simulink model "fixed_point_pi_local_q"  (R2023b)
settings: Solver=FixedStepDiscrete  StartTime=0.0  StopTime=0.02  FixedStep=5.0000000000000002e-05  RelTol=1e-3
values from neighbouring files (symbols this model uses):
  Ki_dt_local = Ki_local * Ts    (= 0.005)    [build_fixed_point_pi_local_q_model.m]
  Kp_local = 10    [build_fixed_point_pi_local_q_model.m]
  Ts = 0.00005    (= 5e-05)    [build_fixed_point_pi_local_q_model.m]    (also in build_fixed_point_pi_q14_model.m)
  Umax_local = 1.8    [build_fixed_point_pi_local_q_model.m]
  Umin_local = -1.8    [build_fixed_point_pi_local_q_model.m]
settings Model: Creator=user  LastModifiedBy=user
settings OptimizationCC: DefaultParameterBehavior=Inlined  EnhancedBackFolding=on  PassReuseOutputArgsAs=Individual arguments  ZeroExternalMemoryAtStartup=off  ZeroInternalMemoryAtStartup=off  OptimizeBlockOrder=speed  DifferentSizesBufferReuse=on  OptimizationCustomize=off  EfficientTunableParamExpr=on
settings DebuggingCC: ParameterTunabilityLossMsg=error
settings HardwareCC: ProdBitPerPointer=32  ProdBitPerSizeT=32  ProdBitPerPtrDiffT=32  ProdLargestAtomicInteger=Long  ProdLargestAtomicFloat=Double  ProdWordSize=32  ProdHWDeviceType=ARM Compatible->ARM Cortex  TargetLargestAtomicInteger=Long  TargetLargestAtomicFloat=Double  TargetIntDivRoundTo=Zero  TargetEndianess=LittleEndian  TargetHWDeviceType=ARM Compatible->ARM Cortex  ProdEqTarget=off
settings SFSimCC: MATLABDynamicMemAlloc=off
settings RTWCC: Description=Embedded Coder  SystemTargetFile=ert.tlc  GenCodeOnly=on  TemplateMakefile=ert_default_tmf  GenerateReport=on
settings CodeAppCC: ForceParamTrailComments=on  IgnoreCustomStorageClasses=off  OperatorAnnotations=on  SimulinkDataObjDesc=on  SFDataObjDesc=on  InsertBlockDesc=on
settings ERTTargetCC: TargetLangStandard=C99 (ISO)  GenerateSampleERTMain=on  InlinedParameterPlacement=NonHierarchical  ERTCustomFileTemplate=example_file_process.tlc

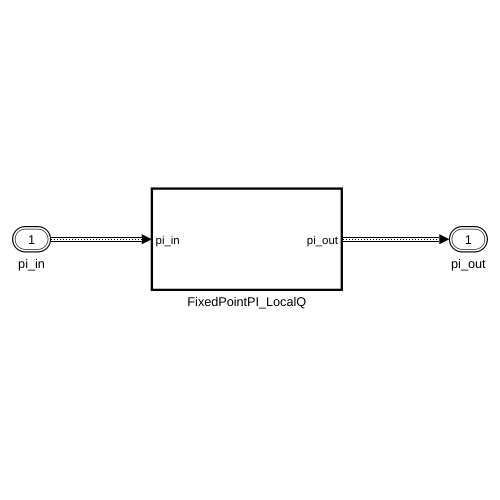
[thumbnail: Simulink's stored preview of the top-level diagram]
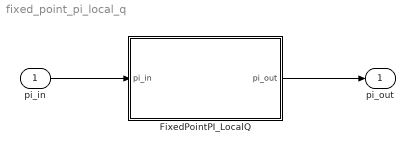
== system fixed_point_pi_local_q ==
  pi_in : Inport  OutDataTypeStr=Bus: FixedPointPI_LocalQ_Input  BusOutputAsStruct=on
  FixedPointPI_LocalQ : Subsystem  TreatAsAtomicUnit=on
  pi_out : Outport  OutDataTypeStr=Bus: FixedPointPI_LocalQ_Output
  wires:
  pi_in/1 -> FixedPointPI_LocalQ/1(pi_in)
  FixedPointPI_LocalQ/1(pi_out) -> pi_out/1

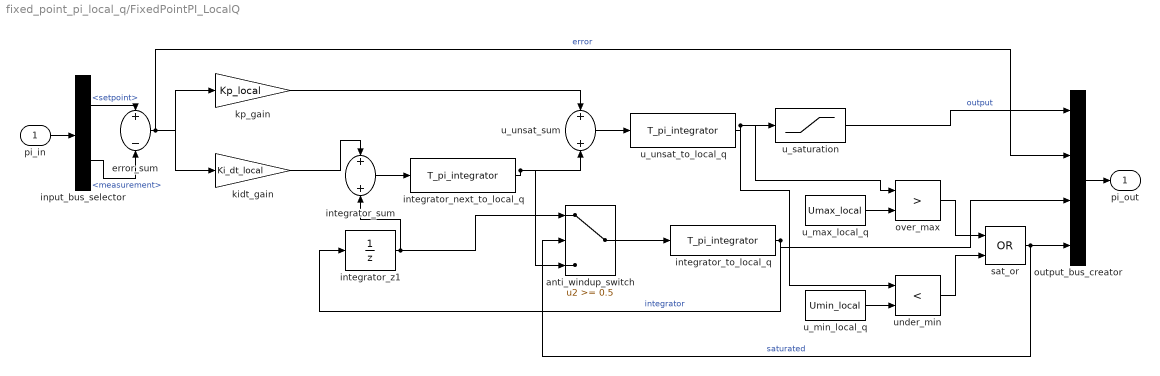
== system fixed_point_pi_local_q/FixedPointPI_LocalQ ==
  pi_in : Inport  OutDataTypeStr=Bus: FixedPointPI_LocalQ_Input  BusOutputAsStruct=on
  anti_windup_switch : Switch  Threshold=0.5  SaturateOnIntegerOverflow=off  InputSameDT=off
  error_sum : Sum  Inputs=+-  OutDataTypeStr=T_pi_io  AccumDataTypeStr=T_pi_integrator  SaturateOnIntegerOverflow=on
  input_bus_selector : BusSelector  OutputSignals=setpoint,measurement
  integrator_next_to_local_q : DataTypeConversion  OutDataTypeStr=T_pi_integrator  RndMeth=Floor
  integrator_sum : Sum  OutDataTypeStr=T_pi_integrator  AccumDataTypeStr=T_pi_integrator  SaturateOnIntegerOverflow=on
  integrator_to_local_q : DataTypeConversion  OutDataTypeStr=T_pi_integrator  RndMeth=Floor
  integrator_z1 : UnitDelay  SampleTime=Ts  HasFrameUpgradeWarning=on
  kidt_gain : Gain  Gain=Ki_dt_local  ParamDataTypeStr=T_pi_gain  OutDataTypeStr=T_pi_integrator  SaturateOnIntegerOverflow=on
  kp_gain : Gain  Gain=Kp_local  ParamDataTypeStr=T_pi_gain  OutDataTypeStr=T_pi_integrator  SaturateOnIntegerOverflow=on
  output_bus_creator : BusCreator  Inputs=4  OutDataTypeStr=Bus: FixedPointPI_LocalQ_Output  NonVirtualBus=on
  over_max : RelationalOperator  Operator=>  OutDataTypeStr=boolean  RndMeth=Simplest  InputSameDT=off
  sat_or : Logic  Operator=OR  AllPortsSameDT=off  OutDataTypeStr=boolean
  u_max_local_q : Constant  Value=Umax_local  OutDataTypeStr=T_pi_integrator
  u_min_local_q : Constant  Value=Umin_local  OutDataTypeStr=T_pi_integrator
  u_saturation : Saturate  UpperLimit=Umax_local  LowerLimit=Umin_local  OutDataTypeStr=T_pi_io
  u_unsat_sum : Sum  OutDataTypeStr=T_pi_integrator  AccumDataTypeStr=T_pi_integrator  SaturateOnIntegerOverflow=on
  u_unsat_to_local_q : DataTypeConversion  OutDataTypeStr=T_pi_integrator  RndMeth=Floor
  under_min : RelationalOperator  Operator=<  OutDataTypeStr=boolean  RndMeth=Simplest  InputSameDT=off
  pi_out : Outport  OutDataTypeStr=Bus: FixedPointPI_LocalQ_Output
  wires:
  pi_in/1 -> input_bus_selector/1
  input_bus_selector/1 -> error_sum/1  "<setpoint>"
  input_bus_selector/2 -> error_sum/2  "<measurement>"
  error_sum/1 -> kp_gain/1, kidt_gain/1, output_bus_creator/2  "error"
  kidt_gain/1 -> integrator_sum/1
  integrator_z1/1 -> integrator_sum/2, anti_windup_switch/1
  integrator_sum/1 -> integrator_next_to_local_q/1
  kp_gain/1 -> u_unsat_sum/1
  integrator_next_to_local_q/1 -> u_unsat_sum/2, anti_windup_switch/3
  u_unsat_sum/1 -> u_unsat_to_local_q/1
  u_unsat_to_local_q/1 -> u_saturation/1, over_max/1, under_min/1
  u_max_local_q/1 -> over_max/2
  u_min_local_q/1 -> under_min/2
  over_max/1 -> sat_or/1
  under_min/1 -> sat_or/2
  sat_or/1 -> anti_windup_switch/2, output_bus_creator/4  "saturated"
  anti_windup_switch/1 -> integrator_to_local_q/1
  integrator_to_local_q/1 -> integrator_z1/1, output_bus_creator/3  "integrator"
  u_saturation/1 -> output_bus_creator/1  "output"
  output_bus_creator/1 -> pi_out/1
